simulink model "New_thermal_conductivity"  (R2013b)
settings: Solver=FixedStepDiscrete  StartTime=0.0  StopTime=10  FixedStep=1  RelTol=1e-3
libraries: carnot x1
settings Model: Creator=awohlfei  LastModifiedBy=awohlfei
settings OptimizationCC: ExpressionDepthLimit=2147483647
settings DebuggingCC: UnderspecifiedInitializationDetection=Simplified  MergeDetectMultiDrivingBlocksExec=error  StateNameClashWarn=warning

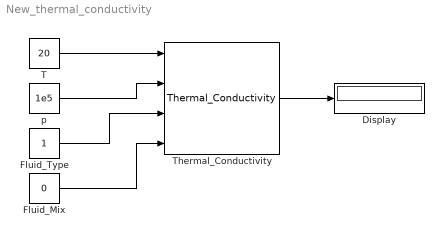
== system New_thermal_conductivity ==
  Display : Display
  Fluid_Mix : Constant  Value=0
  Fluid_Type : Constant
  T : Constant  Value=20
  Thermal_Conductivity : carnot/Basic/Material_Properties/Thermal_Conductivity  VariantControl=CarlibClassic  INPUTARGUMENTS=state variables (classic)  DEBUGLEVEL=WARNINGLEVEL  MAXTOTALMESSAGES=inf  MAXCONSECUTIVEMESSAGES=inf  WRITETOFILE=0  FILENAME='errors.txt'
  p : Constant  Value=1e5
  wires:
  T/1 -> Thermal_Conductivity/1
  p/1 -> Thermal_Conductivity/2
  Fluid_Type/1 -> Thermal_Conductivity/3
  Fluid_Mix/1 -> Thermal_Conductivity/4
  Thermal_Conductivity/1 -> Display/1
